simulink model "Nieliniowy"  (R2012b)
settings: Solver=ode45  StartTime=0.0  StopTime=200  RelTol=1e-3  AbsTol=1e-6
values from neighbouring files (symbols this model uses):
  A1 = 3500    [ZbiorniczkiDokladne.m]
  A2 = 2000    [ZbiorniczkiDokladne.m]
  Aw1 = 0.1 * A1    (= 350)    [ZbiorniczkiDokladne.m]
  Aw2 = 0.1 * A2    (= 200)    [ZbiorniczkiDokladne.m]
  df1 = 200    [ZbiorniczkiDokladne.m]
  f1 = wektorf1(i)    [ZbiorniczkiDokladne.m]
  g = 10    [ZbiorniczkiDokladne.m]
  h1 = ((f1.^2)/((Aw1.^2)*2*g))+((f1+f2).^2)/((Aw2.^2)*2*g)    [ZbiorniczkiDokladne.m]
  h2 = ((f1+f2).^2)/((Aw2.^2)*2*g)    [ZbiorniczkiDokladne.m]
  t1 = 40    [ZbiorniczkiDokladne.m]
settings Model: Creator=LAB320-1552  LastModifiedBy=luki9
settings OptimizationCC: ExpressionDepthLimit=128
settings DebuggingCC: SolverPrmCheckMsg=none  FrameProcessingCompatibilityMsg=error  StrictBusMsg=ErrorOnBusTreatedAsVector
settings CodeAppCC: CustomSymbolStrType=$N$R$M_T
settings GRTTargetCC: CodeReplacementLibrary=C89/C90 (ANSI)

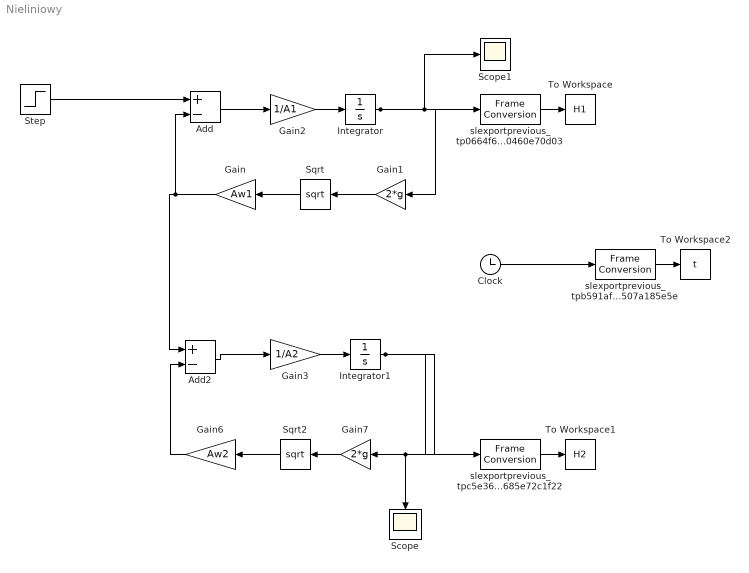
== system Nieliniowy ==
  Add : Sum  Inputs=+-
  Add2 : Sum  Inputs=+-
  Clock : Clock
  Gain : Gain  Gain=Aw1
  Gain1 : Gain  Gain=2*g
  Gain2 : Gain  Gain=1/A1
  Gain3 : Gain  Gain=1/A2
  Gain6 : Gain  Gain=Aw2
  Gain7 : Gain  Gain=2*g
  Integrator : Integrator  InitialCondition=h1
  Integrator1 : Integrator  InitialCondition=h2
  Scope : Scope
      settings: TimeRange=auto  LimitDataPoints=on  MaxDataPoints=5000  SaveToWorkspace=off  SaveName=ScopeData  YMin=0.5849  YMax=1.21592  SampleTime=-1  DataFormat=Array
  Scope1 : Scope
      settings: TimeRange=auto  MaxDataPoints=5000  SaveToWorkspace=off  YMin=0.13059  YMax=0.94059  SampleTime=-1
  Sqrt : Sqrt  SaturateOnIntegerOverflow=on
  Sqrt2 : Sqrt  SaturateOnIntegerOverflow=on
  Step : Step  Time=t1  Before=f1  After=f1+df1  SampleTime=0
  To Workspace : ToWorkspace  VariableName=H1  SampleTime=-1
  To Workspace1 : ToWorkspace  VariableName=H2  SampleTime=-1
  To Workspace2 : ToWorkspace  VariableName=t  SampleTime=-1
  slexportprevious_tp0664f67f_cd2d_40cb_a6e1_e20460e70d03 : FrameConversion  OutFrame=Sample-based
  slexportprevious_tpb591afbe_26f6_40a3_a099_00507a185e5e : FrameConversion  OutFrame=Sample-based
  slexportprevious_tpc5e3657a_5c12_49cd_a928_4685e72c1f22 : FrameConversion  OutFrame=Sample-based
  wires:
  Step/1 -> Add/1
  Add/1 -> Gain2/1
  Gain2/1 -> Integrator/1
  Gain1/1 -> Sqrt/1
  Sqrt/1 -> Gain/1
  Gain/1 -> Add/2, Add2/1
  Integrator/1 -> Scope1/1, Gain1/1, slexportprevious_tp0664f67f_cd2d_40cb_a6e1_e20460e70d03/1
  Add2/1 -> Gain3/1
  Gain3/1 -> Integrator1/1
  Integrator1/1 -> Scope/1, Gain7/1, slexportprevious_tpc5e3657a_5c12_49cd_a928_4685e72c1f22/1
  Gain7/1 -> Sqrt2/1
  Sqrt2/1 -> Gain6/1
  Gain6/1 -> Add2/2
  slexportprevious_tp0664f67f_cd2d_40cb_a6e1_e20460e70d03/1 -> To Workspace/1
  slexportprevious_tpc5e3657a_5c12_49cd_a928_4685e72c1f22/1 -> To Workspace1/1
  Clock/1 -> slexportprevious_tpb591afbe_26f6_40a3_a099_00507a185e5e/1
  slexportprevious_tpb591afbe_26f6_40a3_a099_00507a185e5e/1 -> To Workspace2/1
